simulink model "Circuit2_v3_2018b"  (R2018b)
settings: Solver=ode4  StartTime=0.0  StopTime=5  FixedStep=1e-4  RelTol=1e-3
values from neighbouring files (symbols this model uses):
  A_spol = 1/4 * pi * Dspool^2    (= 7.85398163397e-05)    [Circuit2_values.m]
  Be = 1300e6    (= 1300000000)    [Circuit1_load.m]    (also in Circuit2_values.m)
  BeA = 1200e6    (= 1200000000)    [Circuit2_values.m]    (also in Circut3_values.m = 1300000000)
  Cd = 0.7    [Circuit1_load.m]    (also in Circuit2_values.m)
  Dorifice = 2e-2    (= 0.02)    [Circuit1_load.m]    (also in Circuit2_values.m = 0.004)
  Kp = (1.e-3)/(10e5)    (= 1e-09)    [Circuit1_load.m]    (also in Circuit2_values.m; Circut3_values.m)
  pA0 = 1e5    (= 100000)    [Circuit2_values.m]    (also in Circut3_values.m = 7300000)
  pB0 = 1e5    (= 100000)    [Circuit2_values.m]    (also in Circut3_values.m = 700000)
  pp0 = 180e5    (= 18000000)    [Circuit2_values.m]
  pref = 180e5    (= 18000000)    [Circuit1_load.m]    (also in Circuit2_values.m; Circut3_values.m = 17000000)
  rho = 860    [Circuit1_load.m]    (also in Circuit2_values.m; Circut3_values.m)
  tau = 60e-3    (= 0.06)    [Circuit1_load.m]    (also in Circuit2_values.m = 0.03)
  V = 3e-3    (= 0.003)    [Circuit1_load.m]    (also in Circuit2_values.m)
  VA = 5e-4    (= 0.0005)    [Circuit2_values.m]    (also in Circut3_values.m = 0.0015)
undefined symbols (not defined in the file or in its folder): sgn
settings Model: Creator=Janne  LastModifiedBy=Alex

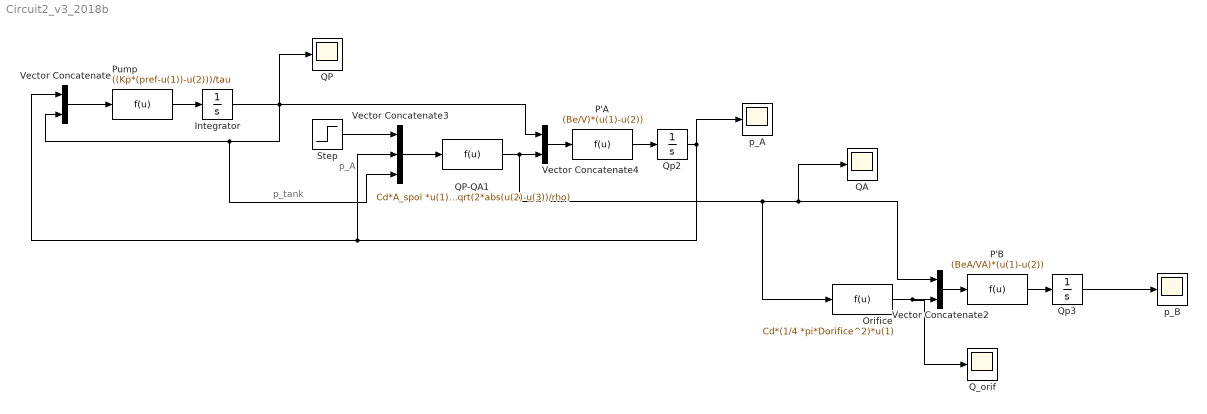
== system Circuit2_v3_2018b ==
  note: p_A
  note: p_tank
  Integrator : Integrator  InitialCondition=pp0  LimitOutput=on  UpperSaturationLimit=1000e5  LowerSaturationLimit=0
  Orifice : Fcn  Expr=Cd*(1/4 *pi*Dorifice^2)*u(1)
  P'A : Fcn  Expr=(Be/V)*(u(1)-u(2))
  P'B : Fcn  Expr=(BeA/VA)*(u(1)-u(2))
  Pump : Fcn  Expr=((Kp*(pref-u(1))-u(2)))/tau
  QA : Scope
  QP : Scope
  QP-QA1 : Fcn  Expr=Cd*A_spol *u(1) * sgn(u(2) - u(3)) *sqrt(2*abs(u(2)-u(3))/rho)
  Q_orif : Scope
  Qp2 : Integrator  InitialCondition=pA0  LimitOutput=on  UpperSaturationLimit=1000e5  LowerSaturationLimit=0
  Qp3 : Integrator  InitialCondition=pB0  LimitOutput=on  UpperSaturationLimit=1000e5  LowerSaturationLimit=0
  Step : Step  Time=2  After=0.0004  SampleTime=0
  Vector Concatenate : Concatenate
  Vector Concatenate2 : Concatenate
  Vector Concatenate3 : Concatenate  NumInputs=3
  Vector Concatenate4 : Concatenate
  p_A : Scope
  p_B : Scope
  wires:
  Pump/1 -> Integrator/1
  Vector Concatenate/1 -> Pump/1
  Vector Concatenate2/1 -> P'B/1
  P'B/1 -> Qp3/1
  Integrator/1 -> QP/1, Vector Concatenate3/3, Vector Concatenate/2, Vector Concatenate4/1
  QP-QA1/1 -> Orifice/1, QA/1, Vector Concatenate2/1, Vector Concatenate4/2
  Vector Concatenate4/1 -> P'A/1
  Vector Concatenate3/1 -> QP-QA1/1
  P'A/1 -> Qp2/1
  Step/1 -> Vector Concatenate3/1
  Qp2/1 -> p_A/1, Vector Concatenate3/2, Vector Concatenate/1
  Orifice/1 -> Q_orif/1, Vector Concatenate2/2
  Qp3/1 -> p_B/1
